simulink model "rccircv2a"  (R2016b)
settings: Solver=VariableStepAuto  StartTime=0.0  StopTime=10.0  RelTol=1e-3
values from neighbouring files (symbols this model uses):
  C = 20000    [rccirc_2a.m]
  R1 = 6.94e-6    (= 6.94e-06)    [rccirc_2a.m]
  tfin = 1e-2    (= 0.01)    [rccirc_2a.m]
  vfin = .04    (= 0.04)    [rccirc_2a.m]
settings Model: Creator=Brian  LastModifiedBy=Brian

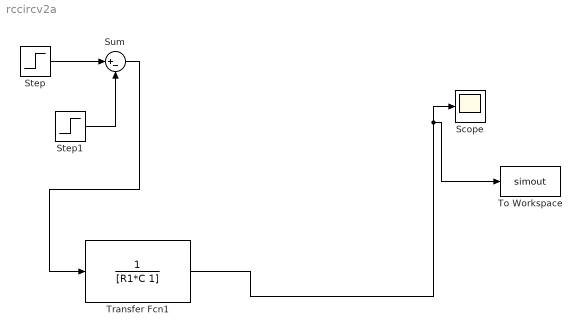
== system rccircv2a ==
  Scope : Scope
  Step : Step  Time=0  After=vfin  SampleTime=0
  Step1 : Step  Time=tfin  After=vfin  SampleTime=0
  Sum : Sum  Inputs=|+-
  To Workspace : ToWorkspace  VariableName=simout  SaveFormat=Timeseries  SampleTime=-1
  Transfer Fcn1 : TransferFcn  Denominator=[R1*C 1]
  wires:
  Sum/1 -> Transfer Fcn1/1
  Step1/1 -> Sum/2
  Step/1 -> Sum/1
  Transfer Fcn1/1 -> To Workspace/1, Scope/1
